simulink model "gm_sampleModel1443_2_sub_sub"  (R2023a)
settings: Solver=VariableStepAuto  StartTime=0.0  StopTime=10.0  RelTol=1e-3
libraries: hdlsllib x4, simulink x1
settings Model: Creator=user1  LastModifiedBy=user1
settings OptimizationCC: BlockReduction=off  ConditionallyExecuteInputs=off
settings DebuggingCC: InheritedTsInSrcMsg=none

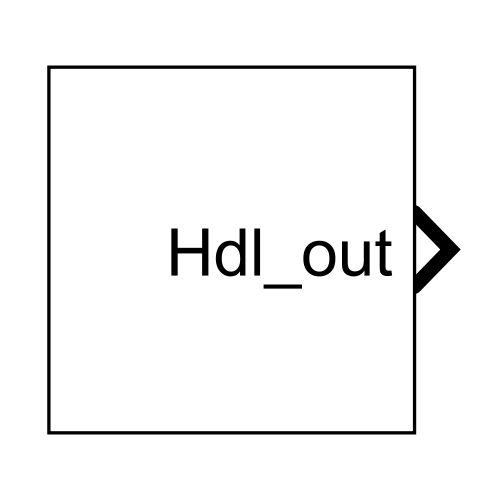
[thumbnail: Simulink's stored preview of the top-level diagram]
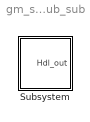
== system gm_sampleModel1443_2_sub_sub ==
  Subsystem : Subsystem

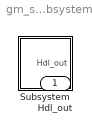
== system gm_sampleModel1443_2_sub_sub/Subsystem ==
  Subsystem : Subsystem
  Hdl_out : Outport  OutDataTypeStr=uint8

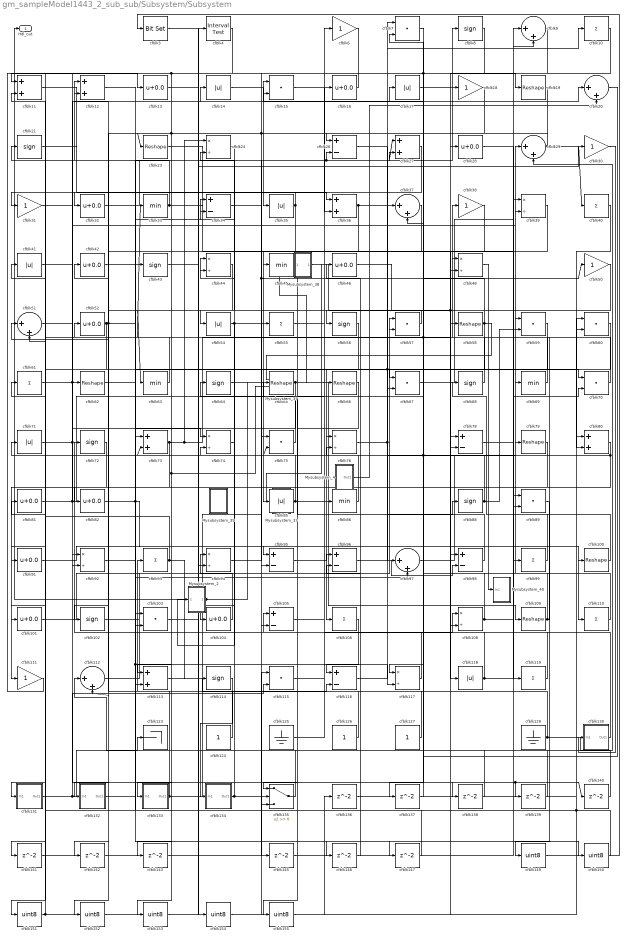
== system gm_sampleModel1443_2_sub_sub/Subsystem/Subsystem ==
  Mysubsystem_2 : Subsystem  TreatAsAtomicUnit=on  RTWFcnName=Mysubsystem_2
      settings: RTWFcnNameOpts=User specified  RTWFileNameOpts=Use function name
  Mysubsystem_33 : Subsystem  TreatAsAtomicUnit=on  RTWFcnName=Mysubsystem_33
      settings: RTWFcnNameOpts=User specified  RTWFileNameOpts=Use function name
  Mysubsystem_37 : Subsystem  TreatAsAtomicUnit=on  RTWFcnName=Mysubsystem_37
      settings: RTWFcnNameOpts=User specified  RTWFileNameOpts=Use function name
  Mysubsystem_38 : Subsystem  TreatAsAtomicUnit=on  RTWFcnName=Mysubsystem_38
      settings: RTWFcnNameOpts=User specified  RTWFileNameOpts=Use function name
  Mysubsystem_39 : Subsystem  TreatAsAtomicUnit=on  RTWFcnName=Mysubsystem_39
      settings: RTWFcnNameOpts=User specified  RTWFileNameOpts=Use function name
  Mysubsystem_4 : Subsystem  TreatAsAtomicUnit=on  RTWFcnName=Mysubsystem_4
      settings: RTWFcnNameOpts=User specified  RTWFileNameOpts=Use function name
  Mysubsystem_40 : Subsystem  TreatAsAtomicUnit=on  RTWFcnName=Mysubsystem_40
      settings: RTWFcnNameOpts=User specified  RTWFileNameOpts=Use function name
  cfblk{10,40,55,61,93,99,106,110,119} (9 alike) : Sum  Inputs=+  OutDataTypeStr=uint8
  cfblk{19,23,58,62,65..66,79,100,109} (9 alike) : Reshape
  cfblk{13,16,28,32,42,46,52,81..82,91,101,104} (12 alike) : Bias  Bias=0.0  SaturateOnIntegerOverflow=off
  cfblk{8,21,43,56,64,68,72,88,102,114} (10 alike) : Signum
  cfblk{7,15,57,59..60,67,70,75,89,103,115} (11 alike) : DotProduct  OutDataTypeStr=uint8
  cfblk{26,34,78,95..96,98,105,116} (8 alike) : Sum  Inputs=+-  OutDataTypeStr=uint8
  cfblk{24,39,44,48,74,76,92,94,108,117} (10 alike) : Product  Inputs=*/  OutDataTypeStr=uint8  RndMeth=Zero  SaturateOnIntegerOverflow=on
  cfblk{11..12,27,36,73,80,113} (7 alike) : Sum  OutDataTypeStr=uint8
  cfblk{6,18,30..31,38,50,111} (7 alike) : Gain  OutDataTypeStr=uint8
  cfblk{9,20,29,37,51,97,112} (7 alike) : Sum  Inputs=|++  OutDataTypeStr=uint8
  cfblk{14,17,35,41,54,71,85,118} (8 alike) : Abs  OutDataTypeStr=uint8  SaturateOnIntegerOverflow=off
  cfblk123 : Terminator
  cfblk124 : Constant  OutDataTypeStr=uint8  SampleTime=-1
  cfblk125 : Ground
  cfblk126 : Constant  OutDataTypeStr=uint8  SampleTime=-1
  cfblk127 : Constant  OutDataTypeStr=uint8  SampleTime=-1
  cfblk129 : Ground
  cfblk130 : Subsystem
      settings: LibrarySourceBlock=|
      | hdlsllib/Ports &
      | Subsystems/Subsystem
  cfblk131 : Subsystem
      settings: LibrarySourceBlock=|
      | hdlsllib/Ports &
      | Subsystems/Subsystem
  cfblk132 : Subsystem
      settings: LibrarySourceBlock=|
      | hdlsllib/Ports &
      | Subsystems/Subsystem
  cfblk133 : Subsystem
      settings: LibrarySourceBlock=|
      | hdlsllib/Ports &
      | Subsystems/Subsystem
  cfblk134 : Subsystem
      settings: LibrarySourceBlock=|
      | hdlsllib/Ports &
      | Subsystems/Subsystem
  cfblk135 : Switch  OutDataTypeStr=uint8  SaturateOnIntegerOverflow=off  InputSameDT=off
  cfblk{136..143,145..147} (11 alike) : Delay  SampleTime=1
  cfblk{149..155} (7 alike) : DataTypeConversion  OutDataTypeStr=uint8  SaturateOnIntegerOverflow=off  RndMeth=Floor
  cfblk3 : simulink/Logic and Bit Operations/Bit Set  iBit=0
      settings: LibrarySourceBlock=|
      | hdlsllib/Logic and Bit
      | Operations/Bit Set
  cfblk{33,45,63,69,86} (5 alike) : MinMax  OutDataTypeStr=uint8
  cfblk4 : hdlsllib/Logic and Bit Operations/Interval Test  IntervalClosedRight=on  uplimit=0.5  IntervalClosedLeft=on  lowlimit=-0.5  OutDataTypeStr=uint8
  Hdl_out : Outport  OutDataTypeStr=uint8
  wires:
  cfblk131/1(Out1) -> cfblk115/2, cfblk123/1
  cfblk65/1 -> cfblk113/2, cfblk109/1
  cfblk72/1 -> cfblk111/1
  cfblk11/1 -> cfblk36/1
  cfblk110/1 -> cfblk29/1
  cfblk111/1 -> cfblk13/1
  cfblk16/1 -> cfblk11/1
  cfblk15/1 -> cfblk36/2
  cfblk10/1 -> cfblk92/2, Mysubsystem_37/2(In2), cfblk143/1
  cfblk9/1 -> cfblk133/1(In1), cfblk23/1
  cfblk4/1 -> cfblk151/1
  cfblk32/1 -> cfblk8/1
  cfblk130/1(Out1) -> cfblk52/1
  cfblk50/1 -> cfblk108/2, cfblk63/1
  cfblk51/1 -> cfblk62/1
  cfblk14/1 -> cfblk35/1
  cfblk129/1 -> cfblk46/1, cfblk29/2
  cfblk52/1 -> cfblk101/1, cfblk112/2, cfblk34/1
  cfblk127/1 -> cfblk44/1
  cfblk30/1 -> cfblk130/1(In1)
  cfblk55/1 -> cfblk16/1
  cfblk35/1 -> cfblk113/1, cfblk32/1
  cfblk124/1 -> cfblk21/1
  cfblk93/1 -> cfblk114/1, cfblk61/1
  cfblk3/1 -> cfblk150/1
  cfblk20/1 -> cfblk117/1
  cfblk135/1 -> cfblk93/1
  cfblk24/1 -> cfblk54/1
  cfblk12/1 -> cfblk70/1
  cfblk106/1 -> cfblk116/1
  cfblk56/1 -> cfblk106/1
  cfblk38/1 -> cfblk85/1
  cfblk134/1(Out1) -> cfblk34/2, cfblk140/1, cfblk139/1
  cfblk39/1 -> cfblk135/1
  cfblk102/1 -> cfblk57/1
  cfblk98/1 -> cfblk65/1
  cfblk69/1 -> cfblk38/1
  cfblk133/1(Out1) -> cfblk51/1, cfblk55/1
  cfblk68/1 -> cfblk17/1, cfblk33/1
  cfblk28/1 -> cfblk119/1
  cfblk117/1 -> cfblk105/1
  cfblk125/1 -> cfblk86/1
  cfblk63/1 -> cfblk42/1
  cfblk79/1 -> cfblk131/1(In1)
  cfblk113/1 -> cfblk116/2
  cfblk33/1 -> cfblk58/1, cfblk12/1
  cfblk67/1 -> cfblk9/1
  cfblk97/1 -> cfblk39/1
  cfblk132/1(Out1) -> cfblk43/1
  cfblk81/1 -> cfblk15/1, cfblk6/1
  cfblk99/1 -> cfblk69/1
  cfblk75/1 -> cfblk44/2
  cfblk119/1 -> cfblk72/1
  cfblk57/1 -> cfblk56/1
  cfblk31/1 -> cfblk14/1
  cfblk91/1 -> cfblk95/1
  cfblk23/1 -> cfblk99/1
  cfblk82/1 -> cfblk110/1, cfblk26/2, cfblk27/1
  cfblk19/1 -> cfblk152/1, cfblk95/2
  cfblk95/1 -> cfblk96/1
  cfblk29/1 -> cfblk26/1, cfblk40/1
  cfblk60/1 -> cfblk76/1
  cfblk21/1 -> cfblk105/2
  cfblk94/1 -> cfblk75/1
  cfblk44/1 -> cfblk132/1(In1)
  cfblk118/1 -> cfblk96/2, cfblk9/2
  cfblk46/1 -> cfblk118/1
  cfblk108/1 -> cfblk64/1, cfblk70/2
  cfblk80/1 -> cfblk103/2, cfblk73/2
  cfblk85/1 -> cfblk74/2, cfblk57/2
  cfblk73/1 -> cfblk102/1, cfblk24/1, cfblk28/1
  cfblk88/1 -> cfblk59/2, cfblk71/1
  cfblk104/1 -> cfblk94/1
  cfblk58/1 -> cfblk7/2, cfblk67/2, cfblk82/1, Mysubsystem_37/1(In1)
  cfblk86/1 -> cfblk11/2
  cfblk105/1 -> cfblk48/1
  cfblk45/1 -> cfblk78/2
  cfblk27/1 -> cfblk91/1
  cfblk62/1 -> cfblk147/1, cfblk117/2
  cfblk17/1 -> cfblk19/1
  cfblk54/1 -> cfblk104/1, cfblk50/1, cfblk27/2
  cfblk71/1 -> cfblk39/2, cfblk92/1
  cfblk116/1 -> cfblk79/1
  cfblk40/1 -> cfblk80/2
  cfblk43/1 -> cfblk30/1
  cfblk41/1 -> cfblk74/1
  cfblk70/1 -> cfblk41/1
  cfblk76/1 -> cfblk100/1, cfblk37/1
  cfblk6/1 -> cfblk31/1
  cfblk36/1 -> cfblk142/1, cfblk10/1
  cfblk78/1 -> cfblk89/1
  cfblk96/1 -> cfblk98/2
  cfblk103/1 -> cfblk135/2
  cfblk34/1 -> cfblk48/2
  cfblk8/1 -> cfblk67/1, cfblk135/3
  cfblk114/1 -> cfblk134/1(In1)
  cfblk126/1 -> cfblk12/2
  cfblk115/1 -> cfblk108/1
  cfblk61/1 -> cfblk138/1, cfblk20/1
  cfblk100/1 -> cfblk68/1
  cfblk26/1 -> cfblk97/1
  cfblk109/1 -> cfblk59/1, cfblk15/2, cfblk75/2
  cfblk112/1 -> cfblk88/1
  cfblk101/1 -> cfblk7/1
  cfblk37/1 -> cfblk45/1
  cfblk92/1 -> cfblk97/2
  cfblk136/1 -> cfblk60/1
  cfblk7/1 -> cfblk137/1
  cfblk137/1 -> cfblk37/2
  cfblk138/1 -> cfblk112/1
  cfblk139/1 -> cfblk73/1
  cfblk140/1 -> cfblk24/2
  cfblk59/1 -> cfblk141/1
  cfblk141/1 -> cfblk94/2
  cfblk142/1 -> cfblk98/1
  cfblk143/1 -> cfblk78/1
  cfblk64/1 -> cfblk145/1
  cfblk145/1 -> cfblk89/2
  cfblk42/1 -> cfblk146/1
  cfblk146/1 -> cfblk76/2
  cfblk147/1 -> cfblk51/2
  cfblk89/1 -> cfblk149/1
  cfblk149/1 -> cfblk3/1
  cfblk150/1 -> cfblk80/1, cfblk103/1
  cfblk151/1 -> cfblk81/1, cfblk115/1
  cfblk152/1 -> cfblk4/1
  cfblk18/1 -> cfblk153/1
  cfblk153/1 -> cfblk136/1
  cfblk13/1 -> cfblk154/1
  cfblk154/1 -> cfblk18/1
  cfblk66/1 -> cfblk155/1
  cfblk155/1 -> cfblk60/2
  cfblk74/1 -> Mysubsystem_2/1(In1)
  Mysubsystem_2/1(Out1) -> Hdl_out/1, cfblk66/1
  Mysubsystem_4/1(Out1) -> cfblk20/2
  Mysubsystem_37/1(Out1) -> Mysubsystem_38/1(In1)
  Mysubsystem_38/1(Out1) -> Mysubsystem_33/1(In1)
  cfblk48/1 -> Mysubsystem_40/1(In1)

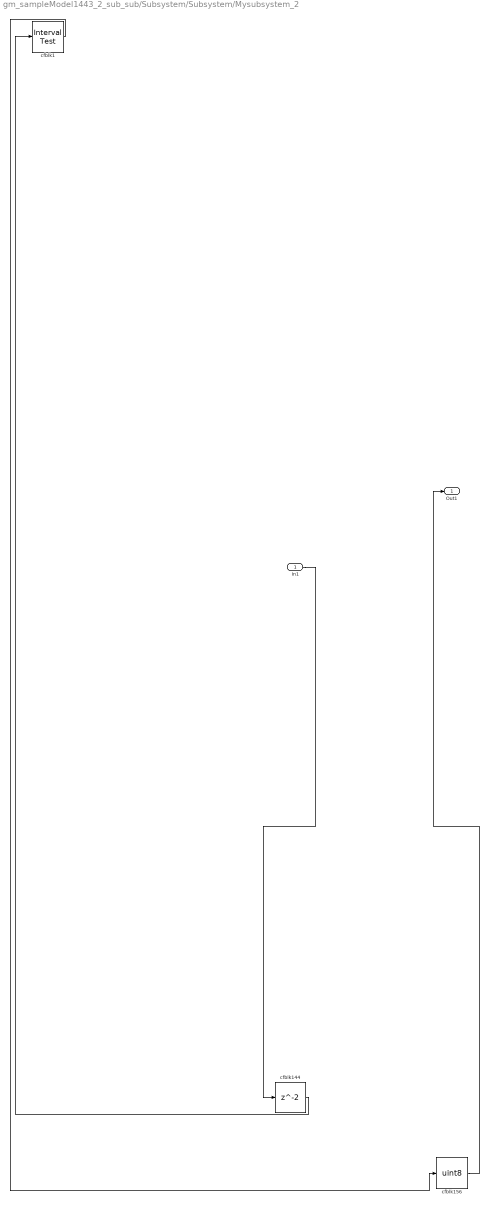
== system gm_sampleModel1443_2_sub_sub/Subsystem/Subsystem/Mysubsystem_2 ==
  In1 : Inport
  cfblk1 : hdlsllib/Logic and Bit Operations/Interval Test  IntervalClosedRight=on  uplimit=0.5  IntervalClosedLeft=on  lowlimit=-0.5  OutDataTypeStr=boolean
  cfblk144 : Delay  SampleTime=1
  cfblk156 : DataTypeConversion  OutDataTypeStr=uint8  SaturateOnIntegerOverflow=off  RndMeth=Floor
  Out1 : Outport
  wires:
  In1/1 -> cfblk144/1
  cfblk144/1 -> cfblk1/1
  cfblk156/1 -> Out1/1
  cfblk1/1 -> cfblk156/1

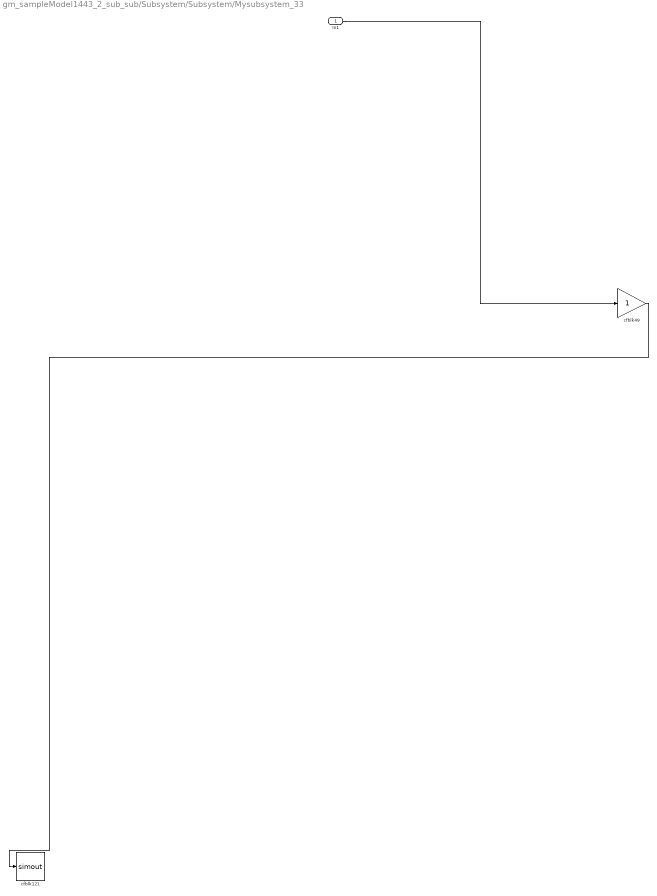
== system gm_sampleModel1443_2_sub_sub/Subsystem/Subsystem/Mysubsystem_33 ==
  In1 : Inport
  cfblk121 : ToWorkspace  VariableName=simout  SaveFormat=Timeseries  SampleTime=-1
  cfblk49 : Gain
  wires:
  In1/1 -> cfblk49/1
  cfblk49/1 -> cfblk121/1

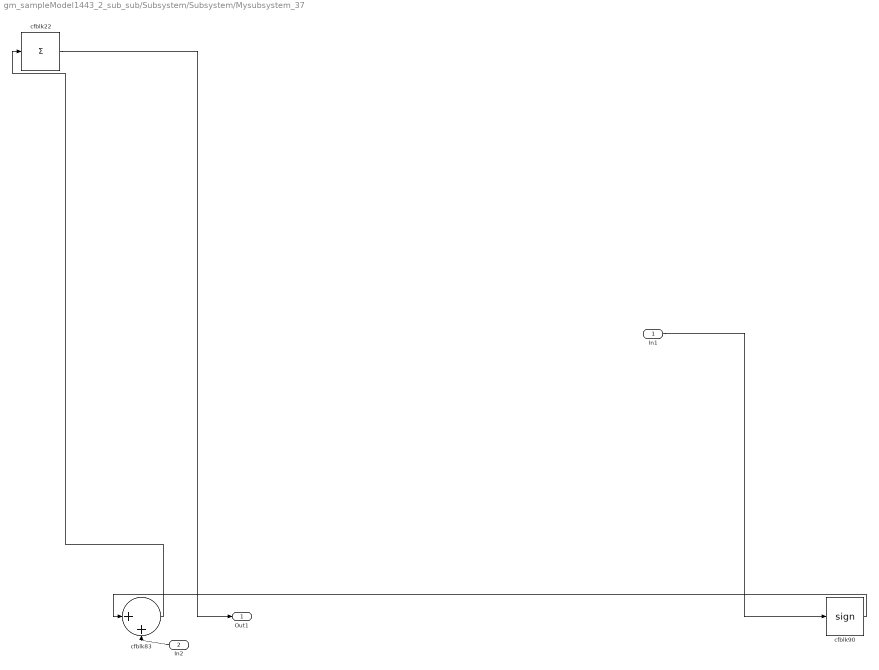
== system gm_sampleModel1443_2_sub_sub/Subsystem/Subsystem/Mysubsystem_37 ==
  In1 : Inport
  In2 : Inport  Port=2
  cfblk22 : Sum  Inputs=+
  cfblk83 : Sum  Inputs=|++
  cfblk90 : Signum
  Out1 : Outport
  wires:
  cfblk22/1 -> Out1/1
  cfblk90/1 -> cfblk83/1
  In1/1 -> cfblk90/1
  cfblk83/1 -> cfblk22/1
  In2/1 -> cfblk83/2

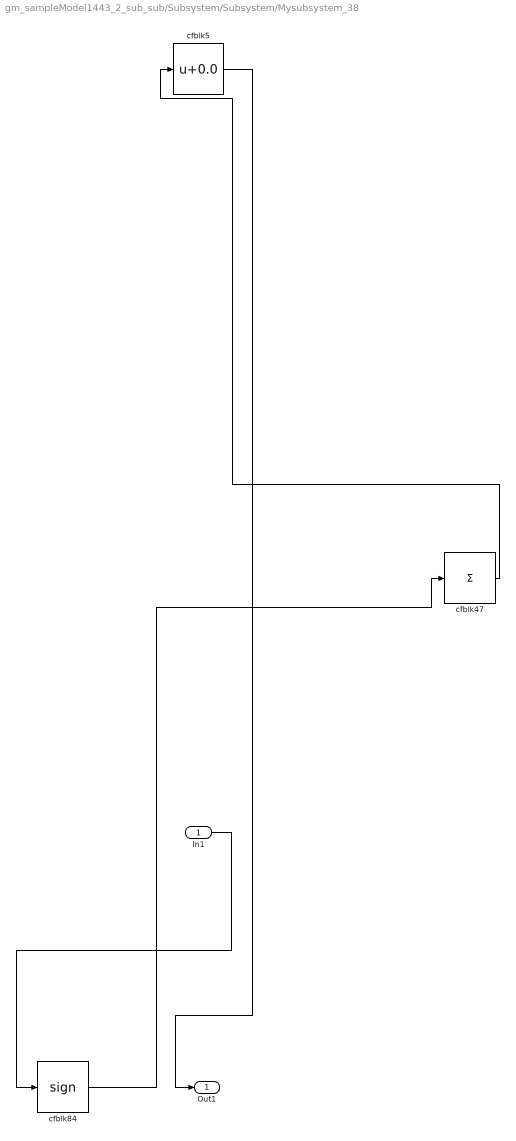
== system gm_sampleModel1443_2_sub_sub/Subsystem/Subsystem/Mysubsystem_38 ==
  In1 : Inport
  cfblk47 : Sum  Inputs=+
  cfblk5 : Bias  Bias=0.0  SaturateOnIntegerOverflow=off
  cfblk84 : Signum
  Out1 : Outport
  wires:
  In1/1 -> cfblk84/1
  cfblk84/1 -> cfblk47/1
  cfblk5/1 -> Out1/1
  cfblk47/1 -> cfblk5/1

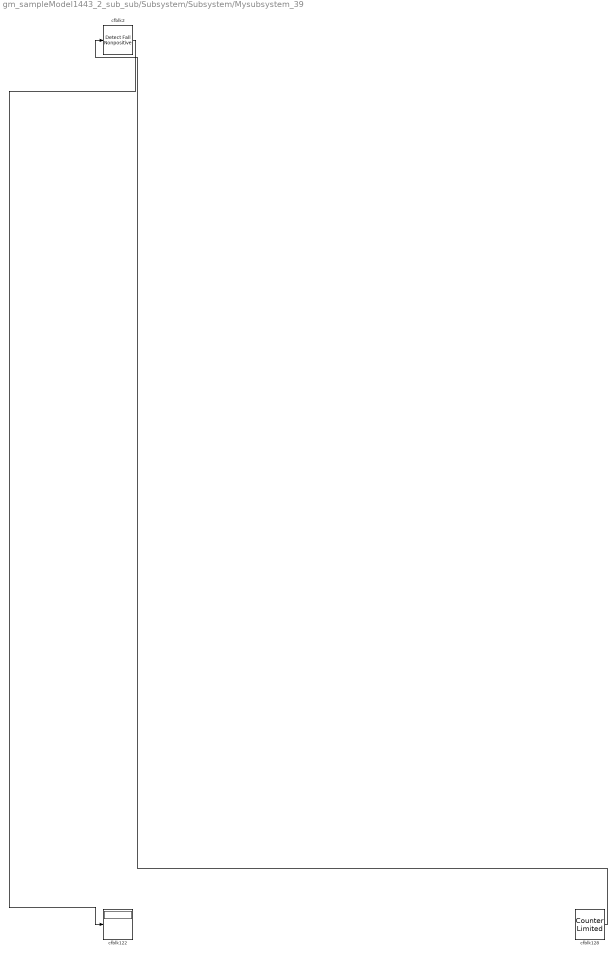
== system gm_sampleModel1443_2_sub_sub/Subsystem/Subsystem/Mysubsystem_39 ==
  cfblk122 : Display
  cfblk128 : hdlsllib/Sources/Counter Limited  uplimit=7  tsamp=-1
  cfblk2 : hdlsllib/Logic and Bit Operations/Detect Fall Nonpositive  vinit=0  OutDataTypeStr=boolean
  wires:
  cfblk2/1 -> cfblk122/1
  cfblk128/1 -> cfblk2/1

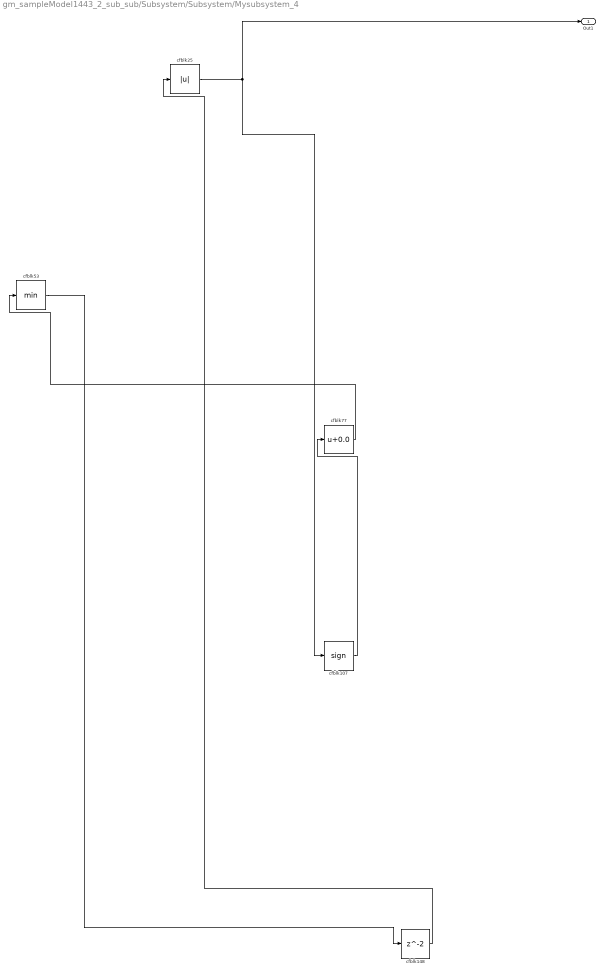
== system gm_sampleModel1443_2_sub_sub/Subsystem/Subsystem/Mysubsystem_4 ==
  cfblk107 : Signum
  cfblk148 : Delay  SampleTime=1
  cfblk25 : Abs  SaturateOnIntegerOverflow=off
  cfblk53 : MinMax
  cfblk77 : Bias  Bias=0.0  SaturateOnIntegerOverflow=off
  Out1 : Outport
  wires:
  cfblk107/1 -> cfblk77/1
  cfblk77/1 -> cfblk53/1
  cfblk25/1 -> cfblk107/1, Out1/1
  cfblk53/1 -> cfblk148/1
  cfblk148/1 -> cfblk25/1

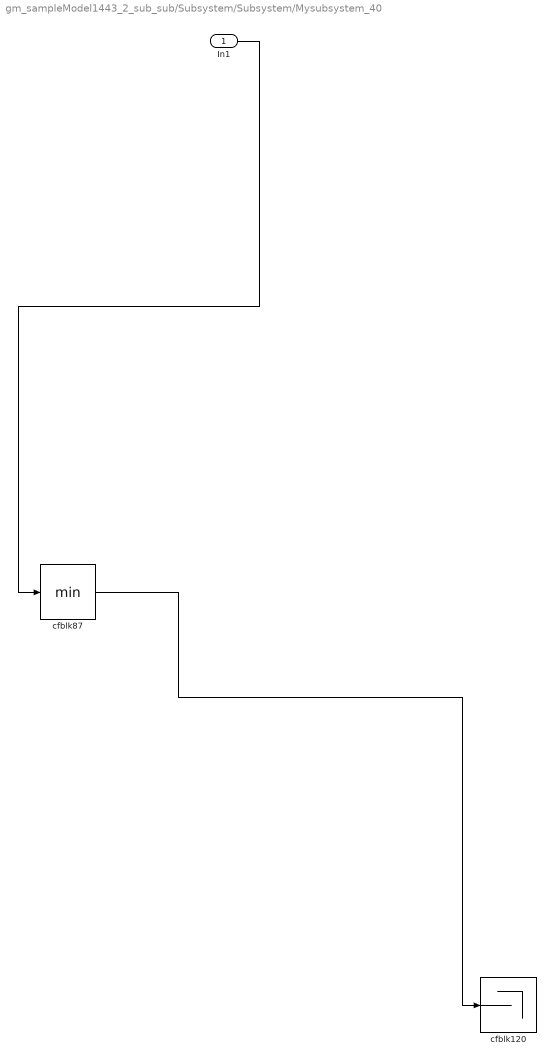
== system gm_sampleModel1443_2_sub_sub/Subsystem/Subsystem/Mysubsystem_40 ==
  In1 : Inport
  cfblk120 : Terminator
  cfblk87 : MinMax
  wires:
  cfblk87/1 -> cfblk120/1
  In1/1 -> cfblk87/1

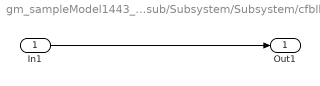
== system gm_sampleModel1443_2_sub_sub/Subsystem/Subsystem/cfblk130 ==
  In1 : Inport
  Out1 : Outport
  wires:
  In1/1 -> Out1/1

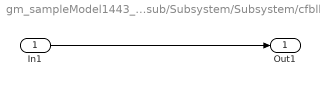
== system gm_sampleModel1443_2_sub_sub/Subsystem/Subsystem/cfblk131 ==
  In1 : Inport
  Out1 : Outport
  wires:
  In1/1 -> Out1/1

== system gm_sampleModel1443_2_sub_sub/Subsystem/Subsystem/cfblk132 ==
  In1 : Inport
  Out1 : Outport
  wires:
  In1/1 -> Out1/1

== system gm_sampleModel1443_2_sub_sub/Subsystem/Subsystem/cfblk133 ==
  In1 : Inport
  Out1 : Outport
  wires:
  In1/1 -> Out1/1

== system gm_sampleModel1443_2_sub_sub/Subsystem/Subsystem/cfblk134 ==
  In1 : Inport
  Out1 : Outport
  wires:
  In1/1 -> Out1/1
